simulink model "test"  (R2014a)
settings: Solver=ode45  StartTime=0.0  StopTime=10.0  RelTol=1e-3
settings Model: Creator=ikemoto  LastModifiedBy=ikemoto

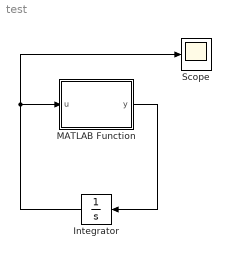
== system test ==
  Integrator : Integrator  InitialCondition=5
  MATLAB Function : MATLAB Function  TreatAsAtomicUnit=on
  Scope : Scope
  wires:
  MATLAB Function/1(y) -> Integrator/1
  Integrator/1 -> Scope/1, MATLAB Function/1(u)

== matlab function test/MATLAB Function ==
  data: u input; y output
function y = fcn(u)
%#codegen

y = testfunc(u);
end
